simulink model "simulacion_completa"  (R2023a)
settings: Solver=VariableStepAuto  StartTime=0.0  StopTime=1  RelTol=1e-3
values from neighbouring files (symbols this model uses):
  filtros = banco_decodificador(Fs, frecuencias_centrales, orden)    [main.m]    (also in sim_falla.m; sim_ideal.m; sim_real.m)
  Fs = 44000    [butter_digital_frec_resp.m]    (also in canal.m; main.m; sim_falla.m; sim_ideal.m)
undefined symbols (not defined in the file or in its folder): f_canal_den, f_canal_num, f_portadora_den, f_portadora_num
libraries: dspstat3 x7, simulink x3
settings Model: Creator=leand  LastModifiedBy=lcampero

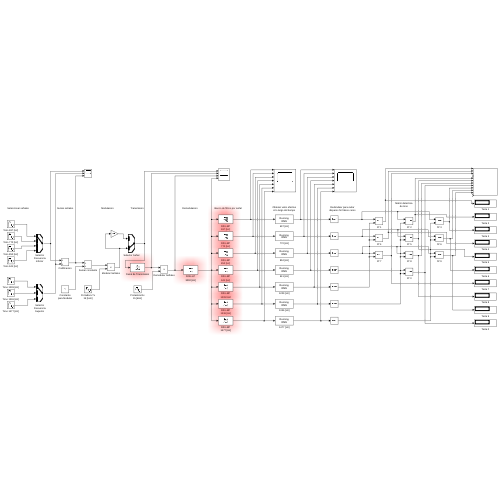
[thumbnail: Simulink's stored preview of the top-level diagram]
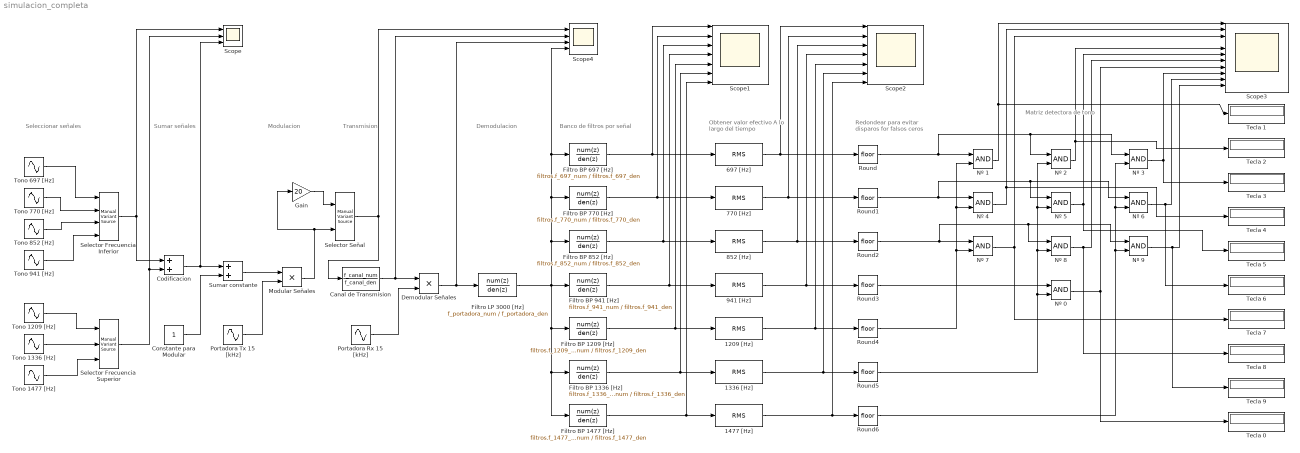
== system simulacion_completa ==
  note: Demodulacion
  note: Transmision
  note: Modulacion
  note: Seleccionar señales
  note: Matriz detectora
      | de tono
  note: Redondear para evitar
      | disparos for falsos ceros
  note: Obtener valor efectivo
      | A lo largo del tiempo
  note: Banco de filtros por señal
  note: Sumar señales
  1209 [Hz] : dspstat3/RMS  run=on  directionMode=Each column  dimension=1  InputProcessing=Columns as channels (frame based)  reset_popup=None
  1336 [Hz] : dspstat3/RMS  run=on  directionMode=Each column  dimension=1  InputProcessing=Columns as channels (frame based)  reset_popup=None
  1477 [Hz] : dspstat3/RMS  run=on  directionMode=Each column  dimension=1  InputProcessing=Columns as channels (frame based)  reset_popup=None
  697 [Hz] : dspstat3/RMS  run=on  directionMode=Entire input  dimension=1  InputProcessing=Columns as channels (frame based)  reset_popup=None
  770 [Hz] : dspstat3/RMS  run=on  directionMode=Each column  dimension=1  InputProcessing=Columns as channels (frame based)  reset_popup=None
  852 [Hz] : dspstat3/RMS  run=on  directionMode=Each column  dimension=1  InputProcessing=Columns as channels (frame based)  reset_popup=None
  941 [Hz] : dspstat3/RMS  run=on  directionMode=Each column  dimension=1  InputProcessing=Columns as channels (frame based)  reset_popup=None
  Canal de Transmision : DiscreteTransferFcn  Numerator=f_canal_num  Denominator=f_canal_den  SampleTime=1/Fs
  Codificacion : Sum
  Constante para Modular : Constant
  Demodular Señales : Product
  Filtro BP 1209 [Hz] : DiscreteTransferFcn  Numerator=filtros.f_1209_num  Denominator=filtros.f_1209_den  SampleTime=1/Fs
  Filtro BP 1336 [Hz] : DiscreteTransferFcn  Numerator=filtros.f_1336_num  Denominator=filtros.f_1336_den  SampleTime=1/Fs
  Filtro BP 1477 [Hz] : DiscreteTransferFcn  Numerator=filtros.f_1477_num  Denominator=filtros.f_1477_den  SampleTime=1/Fs
  Filtro BP 697 [Hz] : DiscreteTransferFcn  Numerator=filtros.f_697_num  Denominator=filtros.f_697_den  SampleTime=1/Fs
  Filtro BP 770 [Hz] : DiscreteTransferFcn  Numerator=filtros.f_770_num  Denominator=filtros.f_770_den  SampleTime=1/Fs
  Filtro BP 852 [Hz] : DiscreteTransferFcn  Numerator=filtros.f_852_num  Denominator=filtros.f_852_den  SampleTime=1/Fs
  Filtro BP 941 [Hz] : DiscreteTransferFcn  Numerator=filtros.f_941_num  Denominator=filtros.f_941_den  SampleTime=1/Fs
  Filtro LP 3000 [Hz] : DiscreteTransferFcn  Numerator=f_portadora_num  Denominator=f_portadora_den  SampleTime=1/Fs
  Gain : Gain  Gain=20
  Modular Señales : Product
  Nº {0..9} (10 alike) : Logic  AllPortsSameDT=off  OutDataTypeStr=boolean
  Portadora Rx 15 [kHz] : Sin  Amplitude=3  Frequency=2*pi*15000  SampleTime=1/Fs
  Portadora Tx 15 [kHz] : Sin  Amplitude=3  Frequency=2*pi*15000  SampleTime=1/Fs
  Round{,1..6} (7 alike) : Rounding
  Scope : Scope  NumInputPorts=3
  Scope1 : Scope  NumInputPorts=7
  Scope2 : Scope  NumInputPorts=7
  Scope3 : Scope  NumInputPorts=12
  Scope4 : Scope  NumInputPorts=4
  Selector Frecuencia Inferior : simulink/Signal Routing/Manual Variant Source  NumChoices=4  LabelModeActiveChoice=V_1
  Selector Frecuencia Superior : simulink/Signal Routing/Manual Variant Source  NumChoices=3  LabelModeActiveChoice=V_1
  Selector Señal : simulink/Signal Routing/Manual Variant Source  NumChoices=2  LabelModeActiveChoice=V_2
  Sumar constante : Sum
  Tecla {0..9} (10 alike) : Display
  Tono 1209 [Hz] : Sin  Frequency=2*pi*1209  SampleTime=1/Fs
  Tono 1336 [Hz] : Sin  Frequency=2*pi*1336  SampleTime=1/Fs
  Tono 1477 [Hz] : Sin  Frequency=2*pi*1477  SampleTime=1/Fs
  Tono 697 [Hz] : Sin  Frequency=2*pi*697  SampleTime=1/Fs
  Tono 770 [Hz] : Sin  Frequency=2*pi*770  SampleTime=1/Fs
  Tono 852 [Hz] : Sin  Frequency=2*pi*852  SampleTime=1/Fs
  Tono 941 [Hz] : Sin  Frequency=2*pi*941  SampleTime=1/Fs
  wires:
  Tono 1209 [Hz]/1 -> Selector Frecuencia Superior/1
  Tono 1336 [Hz]/1 -> Selector Frecuencia Superior/2
  Tono 1477 [Hz]/1 -> Selector Frecuencia Superior/3
  Tono 697 [Hz]/1 -> Selector Frecuencia Inferior/1
  Tono 770 [Hz]/1 -> Selector Frecuencia Inferior/2
  Tono 852 [Hz]/1 -> Selector Frecuencia Inferior/3
  Tono 941 [Hz]/1 -> Selector Frecuencia Inferior/4
  Selector Frecuencia Inferior/1 -> Scope/1, Codificacion/1
  Selector Frecuencia Superior/1 -> Scope/2, Codificacion/2
  Codificacion/1 -> Sumar constante/1, Scope/3
  Filtro BP 770 [Hz]/1 -> 770 [Hz]/1, Scope1/2
  Filtro BP 852 [Hz]/1 -> 852 [Hz]/1, Scope1/3
  Filtro BP 941 [Hz]/1 -> 941 [Hz]/1, Scope1/4
  Filtro BP 1209 [Hz]/1 -> 1209 [Hz]/1, Scope1/5
  Filtro BP 1336 [Hz]/1 -> 1336 [Hz]/1, Scope1/6
  Filtro BP 1477 [Hz]/1 -> 1477 [Hz]/1, Scope1/7
  Filtro BP 697 [Hz]/1 -> 697 [Hz]/1, Scope1/1
  697 [Hz]/1 -> Scope2/1, Round/1
  770 [Hz]/1 -> Round1/1, Scope2/2
  852 [Hz]/1 -> Round2/1, Scope2/3
  941 [Hz]/1 -> Round3/1, Scope2/4
  1209 [Hz]/1 -> Round4/1, Scope2/5
  1336 [Hz]/1 -> Round5/1, Scope2/6
  1477 [Hz]/1 -> Round6/1, Scope2/7
  Round/1 -> Nº 3/1, Nº 2/1, Nº 1/1
  Round1/1 -> Nº 6/1, Nº 5/1, Nº 4/1
  Round2/1 -> Nº 9/1, Nº 8/1, Nº 7/1
  Round3/1 -> Nº 0/1
  Round4/1 -> Nº 7/2, Nº 4/2, Nº 1/2
  Round5/1 -> Nº 8/2, Nº 2/2, Nº 5/2, Nº 0/2
  Round6/1 -> Nº 9/2, Nº 6/2, Nº 3/2
  Nº 1/1 -> Scope3/1, Tecla 1/1
  Nº 4/1 -> Tecla 4/1, Scope3/2
  Nº 7/1 -> Scope3/3, Tecla 7/1
  Nº 2/1 -> Scope3/5, Tecla 2/1
  Nº 5/1 -> Scope3/6, Tecla 5/1
  Nº 8/1 -> Tecla 8/1, Scope3/7
  Nº 0/1 -> Tecla 0/1, Scope3/8
  Nº 3/1 -> Tecla 3/1, Scope3/9
  Nº 6/1 -> Tecla 6/1, Scope3/10
  Nº 9/1 -> Tecla 9/1, Scope3/11
  Constante para Modular/1 -> Sumar constante/2
  Portadora Tx 15 [kHz]/1 -> Modular Señales/2
  Sumar constante/1 -> Modular Señales/1
  Portadora Rx 15 [kHz]/1 -> Demodular Señales/2
  Canal de Transmision/1 -> Scope4/2, Demodular Señales/1
  Demodular Señales/1 -> Scope4/3, Filtro LP 3000 [Hz]/1
  Filtro LP 3000 [Hz]/1 -> Scope4/4, Filtro BP 697 [Hz]/1, Filtro BP 770 [Hz]/1, Filtro BP 852 [Hz]/1, Filtro BP 1477 [Hz]/1, Filtro BP 1336 [Hz]/1, Filtro BP 1209 [Hz]/1, Filtro BP 941 [Hz]/1
  Gain/1 -> Selector Señal/1
  Modular Señales/1 -> Gain/1, Selector Señal/2
  Selector Señal/1 -> Canal de Transmision/1, Scope4/1
